simulink library "LandingGearLibrary"  (R2016a)
settings: Solver=ode45  StartTime=0.0  StopTime=10.0  RelTol=1e-3
values from neighbouring files (symbols this model uses):
  OnOffThreshold = 0.5    [SetConstants.m]
libraries: simulink x5
settings Model: Creator=sj3-wright  LastModifiedBy=Omar
settings DataIOCC: LimitDataPoints=on  SaveFormat=Array
settings DebuggingCC: SolverPrmCheckMsg=warning
settings HardwareCC: ProdBitPerPointer=32  ProdLargestAtomicFloat=None  ProdIntDivRoundTo=Undefined  ProdEndianess=Unspecified  ProdWordSize=32  ProdHWDeviceType=32-bit Generic
settings ModelReferenceCC: PropagateSignalLabelsOutOfModel=off
settings ConfigComp: CovModelRefEnable=Off  CovSFcnEnable=off

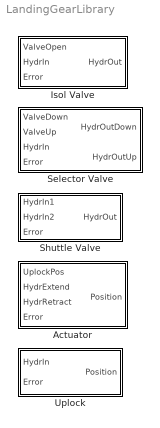
== system LandingGearLibrary ==
  Actuator : Subsystem
  Isol Valve : Subsystem
  Selector Valve : Subsystem
  Shuttle Valve : Subsystem
  Uplock : Subsystem

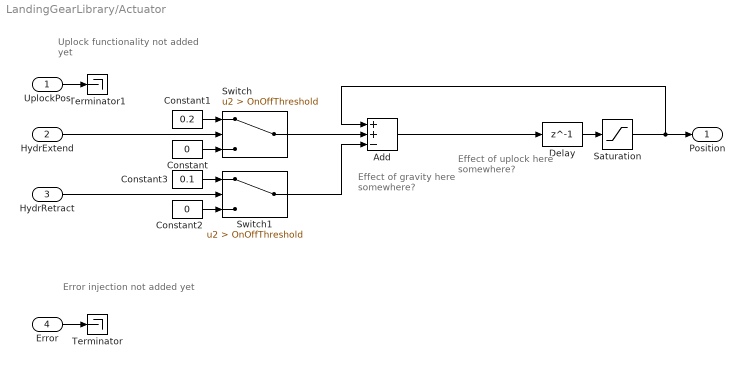
== system LandingGearLibrary/Actuator ==
  note: Uplock functionality
      | not added yet
  note: Error injection
      | not added yet
  note: Effect of
      | uplock
      | here
      | somewhere?
  note: Effect of
      | gravity
      | here
      | somewhere?
  UplockPos : Inport
  HydrExtend : Inport  Port=2
  HydrRetract : Inport  Port=3
  Error : Inport  Port=4
  Add : Sum  Inputs=++-
  Constant : Constant  Value=0
  Constant1 : Constant  Value=0.2
  Constant2 : Constant  Value=0
  Constant3 : Constant  Value=0.1
  Delay : Delay  DelayLength=1  InitialCondition=0
  Saturation : Saturate  UpperLimit=100  LowerLimit=0
  Switch : Switch  Criteria=u2 > Threshold  Threshold=OnOffThreshold
  Switch1 : Switch  Criteria=u2 > Threshold  Threshold=OnOffThreshold
  Terminator : Terminator
  Terminator1 : Terminator
  Position : Outport
  wires:
  Error/1 -> Terminator/1
  UplockPos/1 -> Terminator1/1
  Delay/1 -> Saturation/1
  Saturation/1 -> Add/1, Position/1
  Add/1 -> Delay/1
  Constant/1 -> Switch/3
  HydrExtend/1 -> Switch/2
  Constant1/1 -> Switch/1
  Switch/1 -> Add/2
  HydrRetract/1 -> Switch1/2
  Constant3/1 -> Switch1/1
  Constant2/1 -> Switch1/3
  Switch1/1 -> Add/3

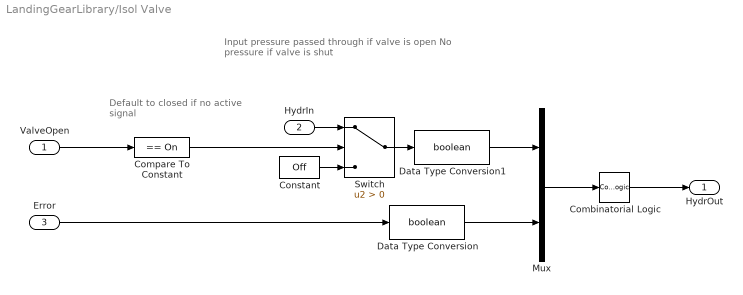
== system LandingGearLibrary/Isol Valve ==
  note: Default to closed if no
      | active signal
  note: Input pressure passed through if valve is open
      | No pressure if valve is shut
  ValveOpen : Inport
  HydrIn : Inport  Port=2
  Error : Inport  Port=3
  Combinatorial Logic : CombinatorialLogic  TruthTable=[0;1;1;0]
  Compare To Constant : simulink/Logic and Bit Operations/Compare To Constant  relop===  const=On  OutDataTypeStr=boolean
  Constant : Constant  Value=Off
  Data Type Conversion : DataTypeConversion  OutDataTypeStr=boolean
  Data Type Conversion1 : DataTypeConversion  OutDataTypeStr=boolean
  Mux : Mux  Inputs=2
  Switch : Switch  Criteria=u2 > Threshold
  HydrOut : Outport
  wires:
  Constant/1 -> Switch/3
  ValveOpen/1 -> Compare To Constant/1
  Compare To Constant/1 -> Switch/2
  HydrIn/1 -> Switch/1
  Mux/1 -> Combinatorial Logic/1
  Combinatorial Logic/1 -> HydrOut/1
  Error/1 -> Data Type Conversion/1
  Switch/1 -> Data Type Conversion1/1
  Data Type Conversion1/1 -> Mux/1
  Data Type Conversion/1 -> Mux/2

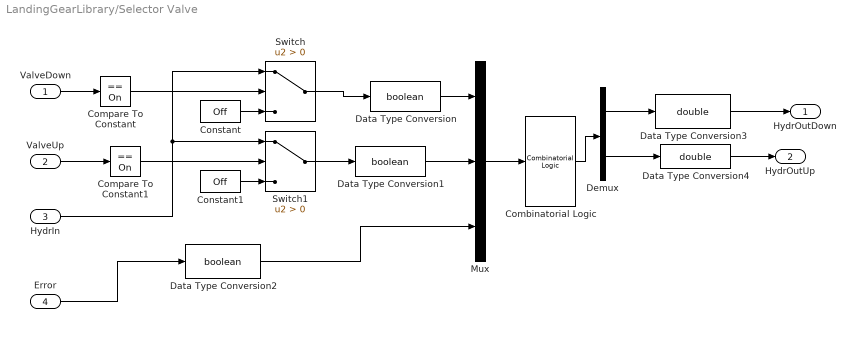
== system LandingGearLibrary/Selector Valve ==
  ValveDown : Inport
  ValveUp : Inport  Port=2
  HydrIn : Inport  Port=3
  Error : Inport  Port=4
  Combinatorial Logic : CombinatorialLogic  TruthTable=[0 0;1 1;0 1;1 0;1 0;0 1;1 1;0 0]
  Compare To Constant : simulink/Logic and Bit Operations/Compare To Constant  relop===  const=On  OutDataTypeStr=boolean
  Compare To Constant1 : simulink/Logic and Bit Operations/Compare To Constant  relop===  const=On  OutDataTypeStr=boolean
  Constant : Constant  Value=Off
  Constant1 : Constant  Value=Off
  Data Type Conversion : DataTypeConversion  OutDataTypeStr=boolean
  Data Type Conversion1 : DataTypeConversion  OutDataTypeStr=boolean
  Data Type Conversion2 : DataTypeConversion  OutDataTypeStr=boolean
  Data Type Conversion3 : DataTypeConversion  OutDataTypeStr=double
  Data Type Conversion4 : DataTypeConversion  OutDataTypeStr=double
  Demux : Demux  Outputs=2
  Mux : Mux  Inputs=3
  Switch : Switch  Criteria=u2 > Threshold
  Switch1 : Switch  Criteria=u2 > Threshold
  HydrOutDown : Outport
  HydrOutUp : Outport  Port=2
  wires:
  Constant/1 -> Switch/3
  Constant1/1 -> Switch1/3
  HydrIn/1 -> Switch1/1, Switch/1
  ValveUp/1 -> Compare To Constant1/1
  ValveDown/1 -> Compare To Constant/1
  Compare To Constant/1 -> Switch/2
  Compare To Constant1/1 -> Switch1/2
  Demux/1 -> Data Type Conversion3/1
  Demux/2 -> Data Type Conversion4/1
  Mux/1 -> Combinatorial Logic/1
  Combinatorial Logic/1 -> Demux/1
  Data Type Conversion/1 -> Mux/1
  Switch/1 -> Data Type Conversion/1
  Switch1/1 -> Data Type Conversion1/1
  Data Type Conversion1/1 -> Mux/2
  Error/1 -> Data Type Conversion2/1
  Data Type Conversion2/1 -> Mux/3
  Data Type Conversion3/1 -> HydrOutDown/1
  Data Type Conversion4/1 -> HydrOutUp/1

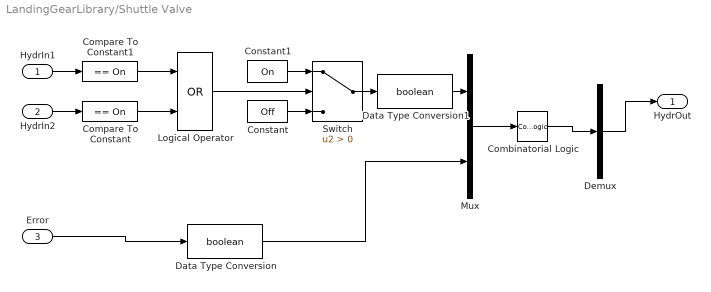
== system LandingGearLibrary/Shuttle Valve ==
  HydrIn1 : Inport
  HydrIn2 : Inport  Port=2
  Error : Inport  Port=3
  Combinatorial Logic : CombinatorialLogic  TruthTable=[0;0;1;0]
  Compare To Constant : simulink/Logic and Bit Operations/Compare To Constant  relop===  const=On  OutDataTypeStr=boolean
  Compare To Constant1 : simulink/Logic and Bit Operations/Compare To Constant  relop===  const=On  OutDataTypeStr=boolean
  Constant : Constant  Value=Off
  Constant1 : Constant  Value=On
  Data Type Conversion : DataTypeConversion  OutDataTypeStr=boolean
  Data Type Conversion1 : DataTypeConversion  OutDataTypeStr=boolean
  Demux : Demux  Outputs=1
  Logical Operator : Logic  Operator=OR  AllPortsSameDT=off  OutDataTypeStr=boolean
  Mux : Mux  Inputs=2
  Switch : Switch  Criteria=u2 > Threshold
  HydrOut : Outport
  wires:
  HydrIn2/1 -> Compare To Constant/1
  HydrIn1/1 -> Compare To Constant1/1
  Compare To Constant/1 -> Logical Operator/2
  Compare To Constant1/1 -> Logical Operator/1
  Constant/1 -> Switch/3
  Logical Operator/1 -> Switch/2
  Constant1/1 -> Switch/1
  Error/1 -> Data Type Conversion/1
  Data Type Conversion/1 -> Mux/2
  Demux/1 -> HydrOut/1
  Switch/1 -> Data Type Conversion1/1
  Data Type Conversion1/1 -> Mux/1
  Combinatorial Logic/1 -> Demux/1
  Mux/1 -> Combinatorial Logic/1

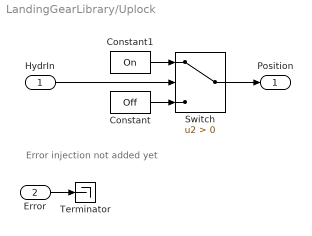
== system LandingGearLibrary/Uplock ==
  note: Error injection
      | not added yet
  HydrIn : Inport
  Error : Inport  Port=2
  Constant : Constant  Value=Off
  Constant1 : Constant  Value=On
  Switch : Switch  Criteria=u2 > Threshold
  Terminator : Terminator
  Position : Outport
  wires:
  Error/1 -> Terminator/1
  Switch/1 -> Position/1
  HydrIn/1 -> Switch/2
  Constant/1 -> Switch/3
  Constant1/1 -> Switch/1
